simulink model "math_functions"  (R2016a)
settings: Solver=VariableStepAuto  StartTime=0.0  StopTime=10.0  RelTol=1e-3
settings Model: Creator=puth  LastModifiedBy=puth

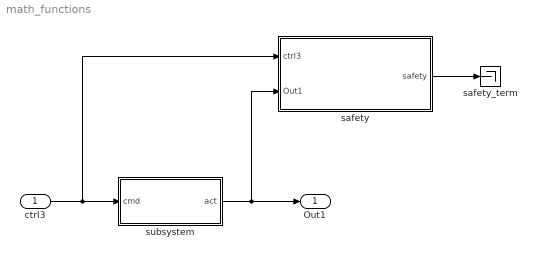
== system math_functions ==
  ctrl3 : Inport
  " subsystem" : Subsystem  RequirementInfo={'other' '..\..\tcm_requirements.docx' '@Simulink_requirement_item_14' 'true' 'Altitude Control' '' } %GIDa_43100e7f_ff6e_4947_8c02_89036f38abbb
  safety : Subsystem  TreatAsAtomicUnit=on  mask(Observer){AnnotationType=ensures, ObserverType=[]}
      mask prompts: AnnotationType "Type of annotation (pre/post...)"; ObserverType "Observer type"
      mask help:
      | Set an observer for the system.
      | The annotation type parameter sets the type of observer:
      | - requires : pre-condition
      | - ensures : post-condition
      | - assert : an assertion
      | - observer : the observer computes a special type of properties
      mask TypeOptions AnnotationType: ensures | requires | assert | observer
      mask Callback AnnotationType:
      | paramStr = get_param(gcb, 'MaskValues');
      | if strcmp(paramStr{1}(1),'o')
      | set_param(gcb,'MaskVisibilities',{'on';'on'});
      | paramStr{2} = 'ellipsoid';
      | set_param(gcb,'MaskValues',paramStr);
      | else
      | set_param(gcb,'MaskVisibilities',{'on';'off'});
      | end
      | clear paramStr;
      mask Callback ObserverType:
      | paramStr = get_param(gcb, 'MaskValues');
      | if strcmp(paramStr{1}(1),'o')
      | set_param(gcb,'MaskVisibilities',{'on';'on'});
      | paramStr{2} = 'ellipsoid';
      | set_param(gcb,'MaskValues',paramStr);
      | else
      | set_param(gcb,'MaskVisibilities',{'on';'off'});
      | end
      | clear paramStr;
      mask Display:
      | color('black')
      | text(0.5, 0.5, ['Property: ''' get_param(gcb,'name') ''''], 'horizontalAlignment', 'center');
      | text(0.99, 0.03, '{\bf\fontsize{12}SAFE}', 'hor', 'right', 'ver', 'bottom', 'texmode', 'on');
  safety_term : Terminator
  Out1 : Outport
  wires:
  safety/1(safety) -> safety_term/1
  ctrl3/1 -> safety/1(ctrl3), " subsystem"/1(cmd)
  " subsystem"/1(act) -> safety/2(Out1), Out1/1

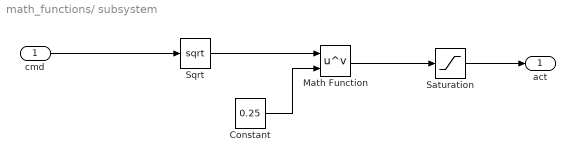
== system math_functions/ subsystem ==
  cmd : Inport
  Constant : Constant  Value=0.25
  Math Function : Math  Operator=pow  SaturateOnIntegerOverflow=on
  Saturation : Saturate  UpperLimit=5  LowerLimit=0
  Sqrt : Sqrt  SaturateOnIntegerOverflow=on
  act : Outport
  wires:
  cmd/1 -> Sqrt/1
  Math Function/1 -> Saturation/1
  Sqrt/1 -> Math Function/1
  Constant/1 -> Math Function/2
  Saturation/1 -> act/1

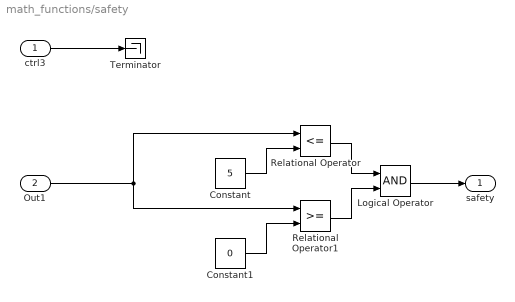
== system math_functions/safety ==
  ctrl3 : Inport
  Out1 : Inport  Port=2
  Constant : Constant  Value=5
  Constant1 : Constant  Value=0
  Logical Operator : Logic  AllPortsSameDT=off  OutDataTypeStr=boolean
  Relational Operator : RelationalOperator  Operator=<=  OutDataTypeStr=boolean
  Relational Operator1 : RelationalOperator  OutDataTypeStr=boolean
  Terminator : Terminator
  safety : Outport
  wires:
  Constant/1 -> Relational Operator/2
  Logical Operator/1 -> safety/1
  Relational Operator/1 -> Logical Operator/1
  Constant1/1 -> Relational Operator1/2
  Relational Operator1/1 -> Logical Operator/2
  Out1/1 -> Relational Operator1/1, Relational Operator/1
  ctrl3/1 -> Terminator/1
